simulink model "PID_Step"  (R2024b)
settings: Solver=FixedStepAuto  StartTime=0.0  StopTime=10.0  FixedStep=0.001  RelTol=1e-3
settings Model: Creator=abdal  LastModifiedBy=abdal

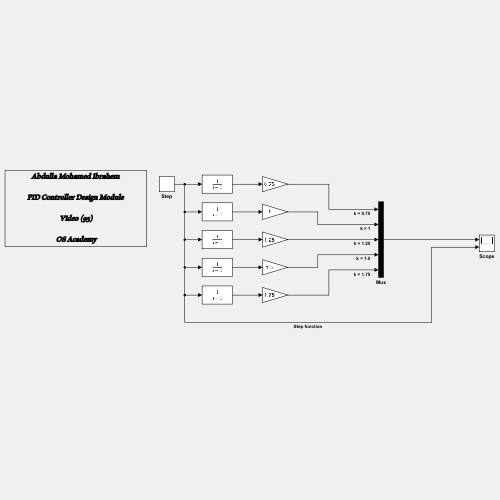
[thumbnail: Simulink's stored preview of the top-level diagram]
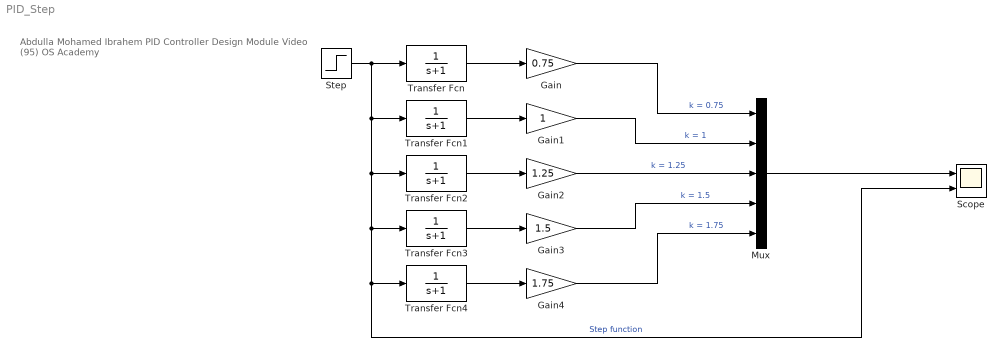
== system PID_Step ==
  note: Abdulla Mohamed Ibrahem
      | PID Controller Design Module
      | Video (95)
      | OS Academy
  Gain : Gain  Gain=0.75
  Gain1 : Gain
  Gain2 : Gain  Gain=1.25
  Gain3 : Gain  Gain=1.5
  Gain4 : Gain  Gain=1.75
  Mux : Mux  Inputs=5
  Scope : Scope  NumInputPorts=2
  Step : Step  SampleTime=0
  Transfer Fcn{,1..4} (5 alike) : TransferFcn  Denominator=[1 1]
  wires:
  Mux/1 -> Scope/1
  Transfer Fcn3/1 -> Gain3/1
  Transfer Fcn/1 -> Gain/1
  Step/1 -> Transfer Fcn4/1, Scope/2, Transfer Fcn3/1, Transfer Fcn2/1, Transfer Fcn1/1, Transfer Fcn/1  "Step function"
  Transfer Fcn1/1 -> Gain1/1
  Transfer Fcn4/1 -> Gain4/1
  Transfer Fcn2/1 -> Gain2/1
  Gain1/1 -> Mux/2  "k = 1"
  Gain3/1 -> Mux/4  "k = 1.5"
  Gain2/1 -> Mux/3  "k = 1.25"
  Gain4/1 -> Mux/5  "k = 1.75"
  Gain/1 -> Mux/1  "k = 0.75"
